simulink model "DC_Motor2"  (R2021b)
settings: Solver=ode23  StartTime=0.0  StopTime=5  MaxStep=1e-5  RelTol=1e-3
libraries: spsDCVoltageSourceLib x2, spsDCMachineLib x1, spsDiodeLib x1, spsGtoLib x1, spsSeriesRLCBranchLib x1, spspowerguiLib x1
settings Model: Creator=win  LastModifiedBy=win

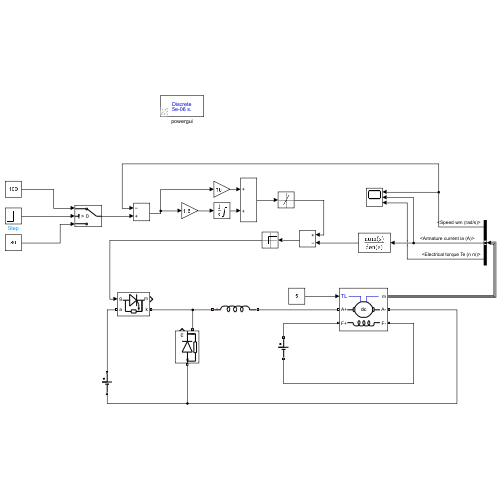
[thumbnail: Simulink's stored preview of the top-level diagram]
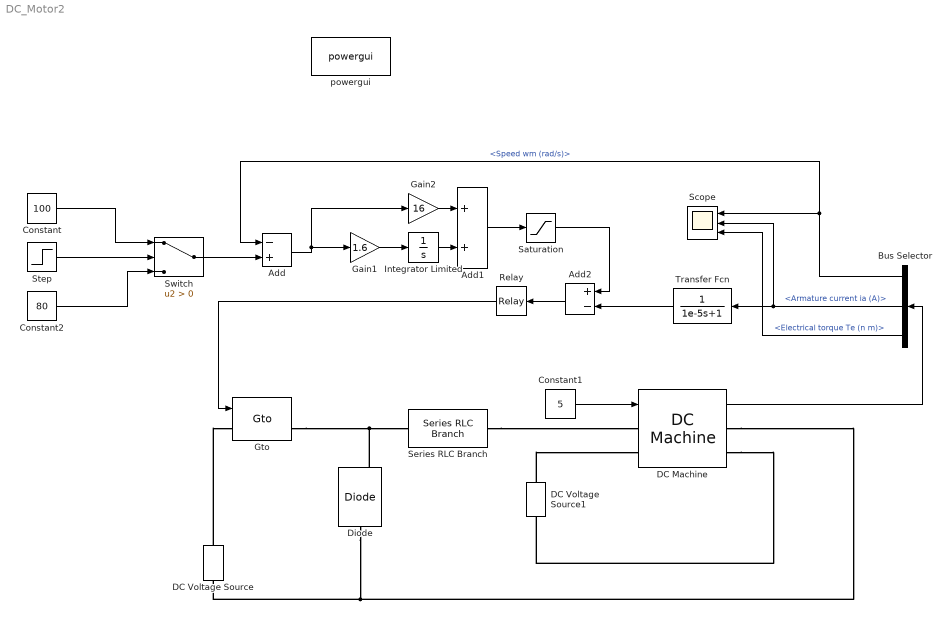
== system DC_Motor2 ==
  Add : Sum  Inputs=-+
  Add1 : Sum
  Add2 : Sum  Inputs=+-
  Bus Selector : BusSelector  OutputSignals=Speed wm (rad/s),Armature current ia (A),Electrical torque Te (n m)
  Constant : Constant  Value=100
  Constant1 : Constant  Value=5
  Constant2 : Constant  Value=80
  DC Machine : spsDCMachineLib/DC Machine  PresetModel=01: 5HP 240V 1750RPM Field:300V  MechanicalLoad=Torque TL  FieldType=Wound  ShowDetailedParameters=on  MeasurementBus=off  RLa=[2.581 0.028]  RLf=[281.2 156]  Laf=0.9483  MachineConstant=Torque constant (N.m/A)  Ke=1.8  Kt=1.8  J=0.02215  Bm=0.002953  Tf=0.5161  w0=1  Ifinit=0.995732574679943  TsPowergui=0  TsBlock=-1
  DC Voltage Source : spsDCVoltageSourceLib/DC Voltage Source  Amplitude=240  Measurements=None
  DC Voltage Source1 : spsDCVoltageSourceLib/DC Voltage Source  Amplitude=280  Measurements=None
  Diode : spsDiodeLib/Diode  Ron=0.001  Lon=0  Vf=0.8  IC=0  UseSnubber=0  Rs=500  Cs=250e-9  Measurements=on
  Gain1 : Gain  Gain=1.6
  Gain2 : Gain  Gain=16
  Gto : spsGtoLib/Gto  Ron=0.001  Lon=0  Vf=1  Tf=10e-6  Tt=20e-6  IC=0  Rs=1e5  Cs=inf  Measurements=on
      settings: SourceProductBaseCode=PS
  Integrator Limited : Integrator  LimitOutput=on  UpperSaturationLimit=+inf
  Relay : Relay
  Saturation : Saturate  UpperLimit=30  LowerLimit=-30
  Scope : Scope  NumInputPorts=3
  Series RLC Branch : spsSeriesRLCBranchLib/Series RLC Branch  LConnTagsString=__new0  RConnTagsString=__new0  BranchType=L  Resistance=1  Inductance=1e-3  SetiL0=off  InitialCurrent=0  Capacitance=1e-6  Setx0=off  InitialVoltage=0  Measurements=None
  Step : Step  SampleTime=0
  Switch : Switch  Criteria=u2 > Threshold
  Transfer Fcn : TransferFcn  Denominator=[1e-5 1]
  powergui : spspowerguiLib/powergui  Priority=1  SimulationMode=Discrete  SampleTime=5e-6  frequency=60  Iterations=50  frequencyindice=0  Pbase=100e6  ErrMax=1e-4  UnitsV=kV  UnitsW=MW  buscounter=0  FunctionMessages=off  echomessages=off  EnableUseOfTLC=off  CurrentSourceSwitches=off  DisableSnubberDevices=off  DisableRonSwitches=off  DisableVfSwitches=off  DisplayEquations=off  AutomaticDiscreteSolvers=off  SolverType=Tustin/Backward Euler (TBE)  Interpol=off  ExternalGateDelay=off  methode=off  Ts=100  x0status=blocks  SPID=on  SwTol=0  HookPort=off  NonlinearTolerance=1e-4  nMaxIteration=100  ContinueOnMaxIteration=off  RestoreLinks=warning  ResistiveCurrentMeasurement=off  Frange=[0:2:500]  Ylog=off  Xlog=on  ShowGrid=off  save=off  variable=ZData  structure=0  ZoomFFT=off  StartTime=0.0  cycles=1  DisplayStyle=1  fundamental=60  FreqAxis=off  MaxFrequency=1000  frequencyindicesteady=1  RmsSteady=1  display=off
  wires:
  DC Machine/1 -> Bus Selector/1
  Bus Selector/1 -> Scope/1, Add/1  "<Speed wm (rad/s)>"
  Add/1 -> Gain2/1, Gain1/1
  Gain1/1 -> Integrator Limited/1
  Integrator Limited/1 -> Add1/2
  Gain2/1 -> Add1/1
  Add1/1 -> Saturation/1
  Bus Selector/2 -> Scope/2, Transfer Fcn/1  "<Armature current ia (A)>"
  Saturation/1 -> Add2/1
  Transfer Fcn/1 -> Add2/2
  Add2/1 -> Relay/1
  Relay/1 -> Gto/1
  Constant1/1 -> DC Machine/1
  Bus Selector/3 -> Scope/3  "<Electrical torque Te (n m)>"
  Step/1 -> Switch/2
  Constant2/1 -> Switch/3
  Switch/1 -> Add/2
  Constant/1 -> Switch/1
  connections:
  DC Voltage Source1/RConn1 -- DC Machine/LConn2
  DC Machine/RConn1 -- Diode/LConn1 -- DC Voltage Source/LConn1
  DC Machine/RConn2 -- DC Voltage Source1/LConn1
  Series RLC Branch/RConn1 -- DC Machine/LConn1
  Diode/RConn1 -- Series RLC Branch/LConn1 -- Gto/RConn1
  DC Voltage Source/RConn1 -- Gto/LConn1
